simulink model "Proyecto_RAII"  (R2025b)
settings: Solver=VariableStepAuto  StartTime=0.0  StopTime=10  RelTol=1e-3
values from neighbouring files (symbols this model uses):
  K = 204/A    (= 0.399217221135)    [Proyecto_RAII.m]
  T = 0.06    [Proyecto_RAII.m]
  Ts = 1/100    (= 0.01)    [Proyecto_RAII.m]
settings Model: Creator=jadel  LastModifiedBy=Usuario

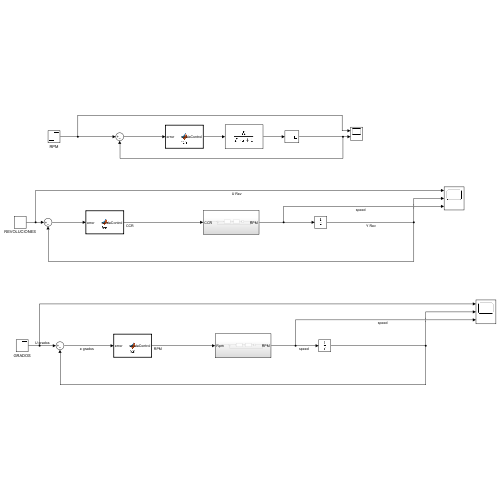
[thumbnail: Simulink's stored preview of the top-level diagram]
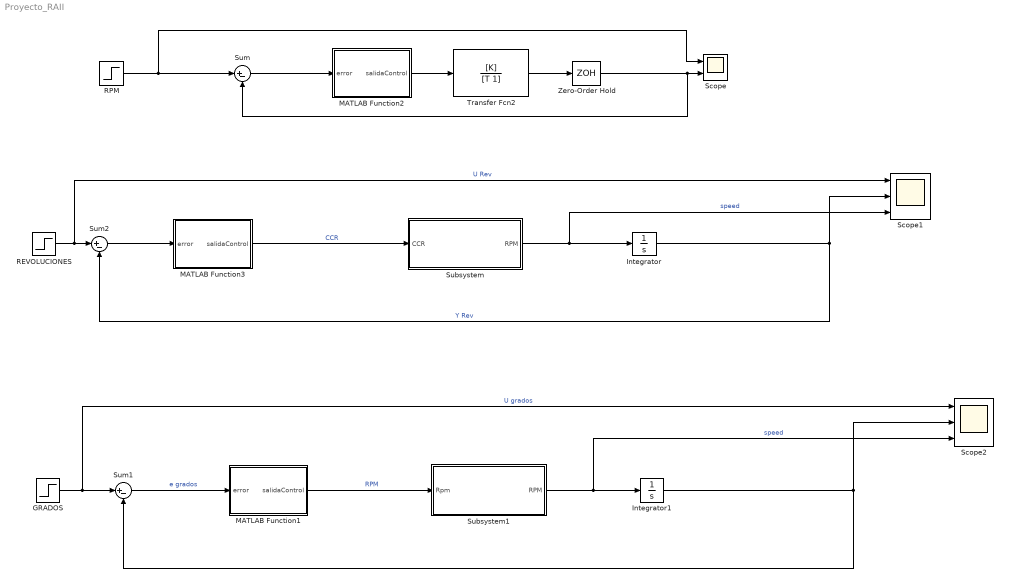
== system Proyecto_RAII ==
  GRADOS : Step  After=90  SampleTime=0
  Integrator : Integrator
  Integrator1 : Integrator
  MATLAB Function1 : MATLAB Function  TreatAsAtomicUnit=on  SystemSampleTime=Ts
  MATLAB Function2 : MATLAB Function  TreatAsAtomicUnit=on  SystemSampleTime=Ts
  MATLAB Function3 : MATLAB Function  TreatAsAtomicUnit=on  SystemSampleTime=Ts
  REVOLUCIONES : Step  Time=0  After=20  SampleTime=0
  RPM : Step  After=300  SampleTime=0
  Scope : Scope  NumInputPorts=2
      settings: ActiveDisplayYMinimum=-37.499999999999993  ActiveDisplayYMaximum=337.5
  Scope1 : Scope  NumInputPorts=3
      settings: ActiveDisplayYMinimum=-23.29992598175955  ActiveDisplayYMaximum=75.049301213463366
  Scope2 : Scope  NumInputPorts=3
      settings: ActiveDisplayYMinimum=-57.100852214643531  ActiveDisplayYMaximum=144.88371511268673  DataLoggingVariableName=ScopeData2
  Subsystem : Subsystem
  Subsystem1 : Subsystem
  Sum : Sum  Inputs=|+-
  Sum1 : Sum  Inputs=|+-
  Sum2 : Sum  Inputs=|+-
  Transfer Fcn2 : TransferFcn  Numerator=[K]  Denominator=[T 1]
  Zero-Order Hold : ZeroOrderHold  SampleTime=Ts
  wires:
  Transfer Fcn2/1 -> Zero-Order Hold/1
  RPM/1 -> Sum/1, Scope/1
  REVOLUCIONES/1 -> Scope1/1, Sum2/1  "U Rev"
  Sum2/1 -> MATLAB Function3/1(error)
  Integrator/1 -> Scope1/2, Sum2/2  "Y Rev"
  MATLAB Function2/1(salidaControl) -> Transfer Fcn2/1
  Sum/1 -> MATLAB Function2/1(error)
  Zero-Order Hold/1 -> Sum/2, Scope/2
  Subsystem/1(RPM) -> Scope1/3, Integrator/1  "speed"
  MATLAB Function3/1(salidaControl) -> Subsystem/1(CCR)  "CCR"
  Subsystem1/1(RPM) -> Scope2/3, Integrator1/1  "speed"
  MATLAB Function1/1(salidaControl) -> Subsystem1/1(Rpm)  "RPM"
  Sum1/1 -> MATLAB Function1/1(error)  "e grados"
  Integrator1/1 -> Scope2/2, Sum1/2
  GRADOS/1 -> Sum1/1, Scope2/1  "U grados"

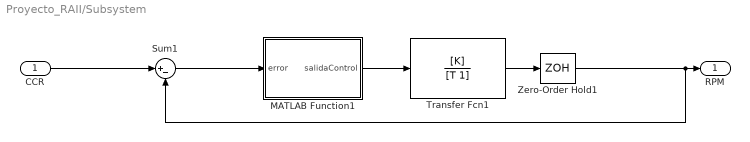
== system Proyecto_RAII/Subsystem ==
  CCR : Inport
  MATLAB Function1 : MATLAB Function  TreatAsAtomicUnit=on  SystemSampleTime=Ts
  Sum1 : Sum  Inputs=|+-
  Transfer Fcn1 : TransferFcn  Numerator=[K]  Denominator=[T 1]
  Zero-Order Hold1 : ZeroOrderHold  SampleTime=Ts
  RPM : Outport
  wires:
  Transfer Fcn1/1 -> Zero-Order Hold1/1
  CCR/1 -> Sum1/1
  Zero-Order Hold1/1 -> Sum1/2, RPM/1
  MATLAB Function1/1(salidaControl) -> Transfer Fcn1/1
  Sum1/1 -> MATLAB Function1/1(error)

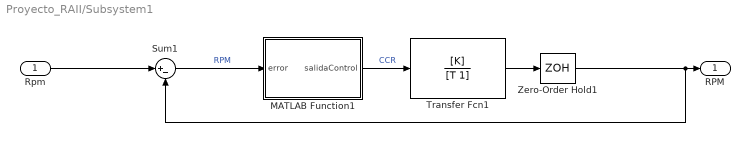
== system Proyecto_RAII/Subsystem1 ==
  Rpm : Inport
  MATLAB Function1 : MATLAB Function  TreatAsAtomicUnit=on  SystemSampleTime=Ts
  Sum1 : Sum  Inputs=|+-
  Transfer Fcn1 : TransferFcn  Numerator=[K]  Denominator=[T 1]
  Zero-Order Hold1 : ZeroOrderHold  SampleTime=Ts
  RPM : Outport
  wires:
  Transfer Fcn1/1 -> Zero-Order Hold1/1
  Rpm/1 -> Sum1/1
  Zero-Order Hold1/1 -> Sum1/2, RPM/1
  MATLAB Function1/1(salidaControl) -> Transfer Fcn1/1  "CCR"
  Sum1/1 -> MATLAB Function1/1(error)  "RPM"

== matlab function Proyecto_RAII/MATLAB Function3 ==
  data: error input; salidaControl output
function salidaControl = fcn(error)
persistent U Y;
if isempty(U)
    U=[0 0];
    Y=[0 0];

end

k= 3.1493;
zero = 0;%0.9563;
U(2)=U(1);
U(1)=error;

Y(2)=Y(1);
Y(1)=k*(U(1)-zero*U(2))+Y(2)*0; % El *0 es por el integrador
% 
% if Y(1)>=40
%     Y(1)=40;
% end
% 
% if (Y(1)-Y(2)>12)
%     Y(1)=Y(2)+12;
% elseif (Y(1)-Y(2)<-12)
%     Y(1)=Y(2)-12;
% end


salidaControl = Y(1);

== matlab function Proyecto_RAII/MATLAB Function2 ==
  data: error input; salidaControl output
function salidaControl = fcn(error)
persistent U Y;
if isempty(U)
    U=[0 0];
    Y=[0 0];

end

k= 1.9665;
zero = 0.7217;
U(2)=U(1);
U(1)=error;

Y(2)=Y(1);
Y(1)=k*(U(1)-zero*U(2))+Y(2);

if (Y(1)>511)
    Y(1)=511;
elseif (Y(1)<-511)
    Y(1)=-511;
end

% if (Y(1)-Y(2)>12)
%     Y(1)=Y(2)+12;
% elseif (Y(1)-Y(2)<-12)
%     Y(1)=Y(2)-12;
% end


salidaControl = Y(1);

== matlab function Proyecto_RAII/MATLAB Function1 ==
  data: error input; salidaControl output
function salidaControl = fcn(error)
persistent U Y;
if isempty(U)
    U=[0 0];
    Y=[0 0];

end

k= 52.48;
zero = 0.9616;
U(2)=U(1);
U(1)=error;

Y(2)=Y(1);
Y(1)=k*(U(1)-zero*U(2))+Y(2)*0; % El *0 es por el integrador

% if Y(1)>=40
%     Y(1)=40;
% end
% 
% if (Y(1)-Y(2)>12)
%     Y(1)=Y(2)+12;
% elseif (Y(1)-Y(2)<-12)
%     Y(1)=Y(2)-12;
% end


salidaControl = Y(1);

== matlab function Proyecto_RAII/Subsystem1/MATLAB Function1 ==
  data: error input; salidaControl output
function salidaControl = fcn(error)
persistent U Y;
if isempty(U)
    U=[0 0];
    Y=[0 0];

end

k= 1.9665;
zero = 0.7217;
U(2)=U(1);
U(1)=error;

Y(2)=Y(1);
Y(1)=k*(U(1)-zero*U(2))+Y(2);

if (Y(1)>511)
    Y(1)=511;
elseif (Y(1)<-511)
    Y(1)=-511;
end

% if (Y(1)-Y(2)>75)
%     Y(1)=Y(2)+75;
% elseif (Y(1)-Y(2)<-75)
%     Y(1)=Y(2)-75;
% end


salidaControl = Y(1);

== matlab function Proyecto_RAII/Subsystem/MATLAB Function1 ==
  data: error input; salidaControl output
function salidaControl = fcn(error)
persistent U Y;
if isempty(U)
    U=[0 0];
    Y=[0 0];

end

k= 1.9665;
zero = 0.7217;
U(2)=U(1);
U(1)=error;

Y(2)=Y(1);
Y(1)=k*(U(1)-zero*U(2))+Y(2);

if (Y(1)>511)
    Y(1)=511;
elseif (Y(1)<-511)
    Y(1)=-511;
end

% if (Y(1)-Y(2)>75)
%     Y(1)=Y(2)+75;
% elseif (Y(1)-Y(2)<-75)
%     Y(1)=Y(2)-75;
% end


salidaControl = Y(1);
